simulink model "Three_phase_AC_Voltage_Controller_R_Load"  (R2023b)
settings: Solver=VariableStepAuto  StartTime=0.0  StopTime=0.06  RelTol=1e-3
undefined symbols (not defined in the file): k
libraries: spsThyristorLib x6, spsACVoltageSourceLib x3, spsSeriesRLCBranchLib x3, spsVoltageMeasurementLib x1, sps_lib x1
settings Model: Creator=HP  LastModifiedBy=HP

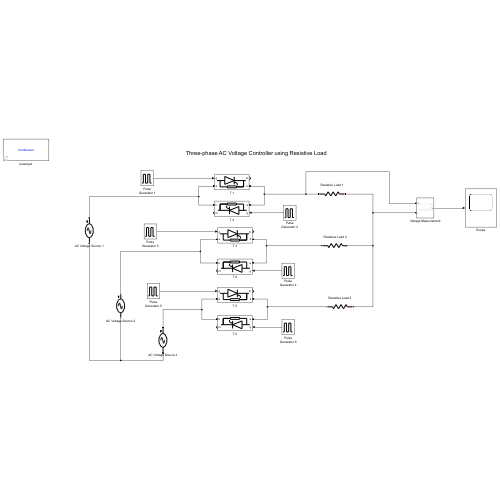
[thumbnail: Simulink's stored preview of the top-level diagram]
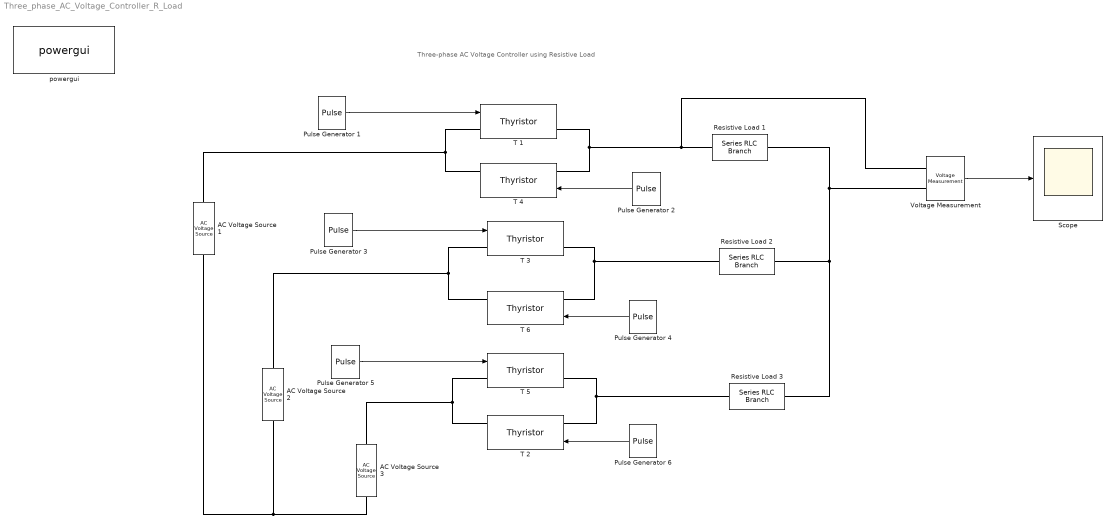
== system Three_phase_AC_Voltage_Controller_R_Load ==
  note: Three-phase AC Voltage Controller using Resistive Load
  AC Voltage Source 1 : spsACVoltageSourceLib/AC Voltage Source  Amplitude=220  Phase=0  Frequency=50  SampleTime=0  Measurements=None  BusType=swing  Pref=10e3  Qref=0  Qmin=-inf  Qmax=+inf
  AC Voltage Source 2 : spsACVoltageSourceLib/AC Voltage Source  Amplitude=220  Phase=-120  Frequency=50  SampleTime=0  Measurements=None  BusType=swing  Pref=10e3  Qref=0  Qmin=-inf  Qmax=+inf
  AC Voltage Source 3 : spsACVoltageSourceLib/AC Voltage Source  Amplitude=220  Phase=120  Frequency=50  SampleTime=0  Measurements=None  BusType=swing  Pref=10e3  Qref=0  Qmin=-inf  Qmax=+inf
  Pulse Generator 1 : DiscretePulseGenerator  PulseType=Time based  Period=0.02  PulseWidth=60  PhaseDelay=k*(0.02/360)
  Pulse Generator 2 : DiscretePulseGenerator  PulseType=Time based  Period=0.02  PulseWidth=60  PhaseDelay=(k+180)*(0.02/360)
  Pulse Generator 3 : DiscretePulseGenerator  PulseType=Time based  Period=0.02  PulseWidth=60  PhaseDelay=(k+120)*(0.02/360)
  Pulse Generator 4 : DiscretePulseGenerator  PulseType=Time based  Period=0.02  PulseWidth=60  PhaseDelay=(k+300)*(0.02/360)
  Pulse Generator 5 : DiscretePulseGenerator  PulseType=Time based  Period=0.02  PulseWidth=60  PhaseDelay=(k+240)*(0.02/360)
  Pulse Generator 6 : DiscretePulseGenerator  PulseType=Time based  Period=0.02  PulseWidth=60  PhaseDelay=(k+60)*(0.02/360)
  Resistive Load 1 : spsSeriesRLCBranchLib/Series RLC Branch  LConnTagsString=__new0  RConnTagsString=__new0  BranchType=R  Resistance=10  Inductance=1e-3  SetiL0=off  InitialCurrent=0  Capacitance=1e-6  Setx0=off  InitialVoltage=0  Measurements=None
  Resistive Load 2 : spsSeriesRLCBranchLib/Series RLC Branch  LConnTagsString=__new0  RConnTagsString=__new0  BranchType=R  Resistance=10  Inductance=1e-3  SetiL0=off  InitialCurrent=0  Capacitance=1e-6  Setx0=off  InitialVoltage=0  Measurements=None
  Resistive Load 3 : spsSeriesRLCBranchLib/Series RLC Branch  LConnTagsString=__new0  RConnTagsString=__new0  BranchType=R  Resistance=10  Inductance=1e-3  SetiL0=off  InitialCurrent=0  Capacitance=1e-6  Setx0=off  InitialVoltage=0  Measurements=None
  Scope : Scope
  T {1..6} (6 alike) : spsThyristorLib/Thyristor  Ron=0.001  Lon=0  Vf=0.8  IC=0  Rs=500  Cs=250e-9  Measurements=on
  Voltage Measurement : spsVoltageMeasurementLib/Voltage Measurement  PhasorSimulation=off  OutputType=Complex  PSBequivalent=0
  powergui : sps_lib/powergui  Priority=1  SimulationMode=Continuous  SampleTime=50e-6  frequency=60  Iterations=50  frequencyindice=50  Pbase=100e6  ErrMax=1e-4  UnitsV=kV  UnitsW=MW  buscounter=0  FunctionMessages=off  echomessages=off  EnableUseOfTLC=off  CurrentSourceSwitches=off  DisableSnubberDevices=off  DisableRonSwitches=off  DisableVfSwitches=off  DisplayEquations=off  AutomaticDiscreteSolvers=off  SolverType=Tustin/Backward Euler (TBE)  Interpol=off  ExternalGateDelay=off  methode=off  Ts=100  x0status=blocks  SPID=on  SwTol=0  HookPort=off  NonlinearTolerance=1e-4  nMaxIteration=100  ContinueOnMaxIteration=off  RestoreLinks=warning  ResistiveCurrentMeasurement=off  Frange=[0:2:500]  Ylog=off  Xlog=on  ShowGrid=off  save=off  variable=ZData  structure=0  ZoomFFT=off  StartTime=0.0  cycles=1  DisplayStyle=1  fundamental=60  FreqAxis=off  MaxFrequency=1000  frequencyindicesteady=1  RmsSteady=1  display=off
  wires:
  Voltage Measurement/1 -> Scope/1
  Pulse Generator 1/1 -> T 1/1
  Pulse Generator 2/1 -> T 4/1
  Pulse Generator 3/1 -> T 3/1
  Pulse Generator 5/1 -> T 5/1
  Pulse Generator 4/1 -> T 6/1
  Pulse Generator 6/1 -> T 2/1
  connections:
  T 1/RConn1 -- Voltage Measurement/LConn1 -- Resistive Load 1/RConn1 -- T 4/LConn1
  T 1/LConn1 -- AC Voltage Source 1/RConn1 -- T 4/RConn1
  T 3/RConn1 -- T 6/LConn1 -- Resistive Load 2/RConn1
  T 3/LConn1 -- AC Voltage Source 2/RConn1 -- T 6/RConn1
  T 5/RConn1 -- Resistive Load 3/RConn1 -- T 2/LConn1
  T 5/LConn1 -- AC Voltage Source 3/RConn1 -- T 2/RConn1
  AC Voltage Source 3/LConn1 -- AC Voltage Source 2/LConn1 -- AC Voltage Source 1/LConn1
  Resistive Load 1/LConn1 -- Voltage Measurement/LConn2 -- Resistive Load 2/LConn1 -- Resistive Load 3/LConn1
